simulink model "ExperimentalLab2Assignments"  (R2020b)
settings: Solver=VariableStepAuto  StartTime=0.0  StopTime=10.0  RelTol=1e-3
undefined symbols (not defined in the file): BEMF_Compensator, Beq_hat_final, C, denCd, DiscIntNeverNeededParam, friction_Compensator, Gamma0, gbox, H0, inertia_Compensator, J0, K, Kd, Ke, Ki, Kp, Kw, National_Instruments, Nu, numCd, Nx, PCIe, Phi0, rpm2rads, sens, stepAmplitude, tau_sf_hat_final, Tl, Ts
libraries: sldrtlib x15, simulink x1
settings Model: Creator=Musta  LastModifiedBy=Musta

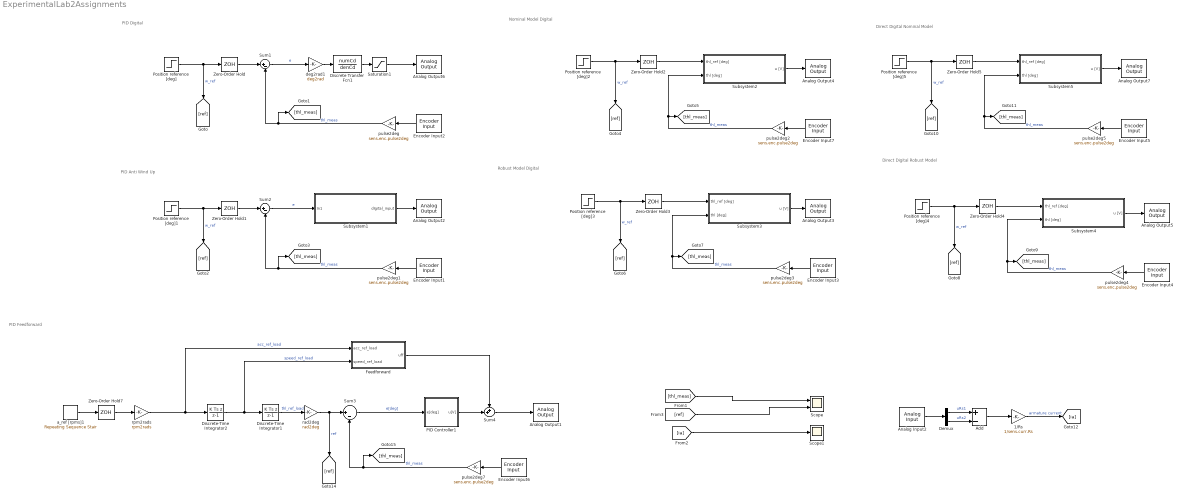
== system ExperimentalLab2Assignments ==
  note: PID Feedforward
  note: Direct Digital Nominal Model
  note: Direct Digital Robust Model
  note: Robust Model Digital
  note: Nominal Model Digital
  note: PID Anti Wind Up
  note: PID Digital
  1/Rs : Gain  Gain=1/sens.curr.Rs
  Add : Sum  Inputs=+-
  Analog Input2 : sldrtlib/Analog Input  SampleTime=0.001  MaxMissedTicks=10  ShowMissedTicks=off  YieldWhenWaiting=off  DrvName=National_Instruments/PCIe-6321  DrvAddress=4294967295  DrvOptions=[0 0 0 2 0 0 0]  Channels=[1,2]  RangeMode=1  VoltRange=1  DataType=1
      settings: AttributesFormatString=National Instruments\nPCIe-6321 [auto]
  Analog Output{1..7} (7 alike) : sldrtlib/Analog Output  SampleTime=0.001  MaxMissedTicks=10  ShowMissedTicks=off  YieldWhenWaiting=off  DrvName=National_Instruments/PCIe-6321  DrvAddress=4294967295  DrvOptions=[0 0 0 2 0 0 0]  Channels=1  RangeMode=1  VoltRange=1  InitialValue=0  FinalValue=0
      settings: AttributesFormatString=National Instruments\nPCIe-6321 [auto]
  Demux : Demux  Outputs=2
  Discrete Transfer Fcn1 : DiscreteTransferFcn  Numerator=numCd  Denominator=denCd  SampleTime=Ts
  Discrete-Time Integrator1 : DiscreteIntegrator  IntegratorMethod=Integration: Backward Euler  SampleTime=Ts  ICPrevOutput=DiscIntNeverNeededParam  ICPrevScaledInput=DiscIntNeverNeededParam
  Discrete-Time Integrator2 : DiscreteIntegrator  IntegratorMethod=Integration: Backward Euler  SampleTime=Ts  ICPrevOutput=DiscIntNeverNeededParam  ICPrevScaledInput=DiscIntNeverNeededParam
  Encoder Input{1..7} (7 alike) : sldrtlib/Encoder Input  SampleTime=0.001  MaxMissedTicks=10  ShowMissedTicks=off  YieldWhenWaiting=off  DrvName=National_Instruments/PCIe-6321  DrvAddress=4294967295  DrvOptions=[0 0 0 2 0 0 0]  Channels=1  QuadMode=3  IndexPulse=2  InputFilter=Inf  DataType=1
      settings: AttributesFormatString=National Instruments\nPCIe-6321 [auto]
  Feedforward : Subsystem
  PID Controller1 : Subsystem
  Position reference [deg]{,1..5} (6 alike) : Step  After=stepAmplitude  SampleTime=0
  Saturation1 : Saturate  UpperLimit=10  LowerLimit=-10
  Scope : Scope  NumInputPorts=2
  Scope1 : Scope
  Subsystem1 : Subsystem
  Subsystem2 : Subsystem
  Subsystem3 : Subsystem
  Subsystem4 : Subsystem
  Subsystem5 : Subsystem
  Sum1 : Sum  Inputs=|+-
  Sum2 : Sum  Inputs=|+-
  Sum3 : Sum  Inputs=|+-
  Sum4 : Sum  Inputs=++|
  Zero-Order Hold{,1..5,7} (7 alike) : ZeroOrderHold  SampleTime=Ts
  a_ref [rpms]1 : simulink/Sources/Repeating Sequence Stair  OutValues=[900 0 -900 -900 0 900].'  tsamp=0.5  OutMin=[]  OutMax=[]  OutDataTypeStr=double  OutputDataTypeScalingMode=double  OutDataType=fixdt(0,8)  ConRadixGroup=Best Precision: Vector-wise  OutScaling=2^-12
  deg2rad1 : Gain  Gain=deg2rad
  pulse2deg{,1..5,7} (7 alike) : Gain  Gain=sens.enc.pulse2deg
  rad2deg : Gain  Gain=rad2deg
  rpm2rads : Gain  Gain=rpm2rads
  wires:
  Zero-Order Hold/1 -> Sum1/1
  Saturation1/1 -> Analog Output6/1
  pulse2deg/1 -> [thl_meas], Sum1/2  "thl_meas"
  Position reference [deg]/1 -> Zero-Order Hold/1, [ref]  "w_ref"
  Encoder Input2/1 -> pulse2deg/1
  Sum1/1 -> deg2rad1/1  "e"
  Subsystem1/1(dIgital_input) -> Analog Output2/1
  Position reference [deg]1/1 -> Zero-Order Hold1/1, [ref]  "w_ref"
  Encoder Input1/1 -> pulse2deg1/1
  pulse2deg1/1 -> [thl_meas], Sum2/2  "thl_meas"
  Zero-Order Hold1/1 -> Sum2/1
  Sum2/1 -> Subsystem1/1(In1)  "e"
  Subsystem2/1(u [V]) -> Analog Output4/1
  Zero-Order Hold2/1 -> Subsystem2/1(thl_ref [deg])
  pulse2deg2/1 -> Subsystem2/2(thl [deg]), [thl_meas]  "thl_meas"
  Encoder Input7/1 -> pulse2deg2/1
  Position reference [deg]2/1 -> [ref], Zero-Order Hold2/1  "w_ref"
  Zero-Order Hold3/1 -> Subsystem3/1(thl_ref [deg])
  Position reference [deg]3/1 -> [ref], Zero-Order Hold3/1  "w_ref"
  Subsystem3/1(u [V]) -> Analog Output3/1
  Encoder Input3/1 -> pulse2deg3/1
  pulse2deg3/1 -> Subsystem3/2(thl [deg]), [thl_meas]  "thl_meas"
  Subsystem4/1(u [V]) -> Analog Output5/1
  Encoder Input4/1 -> pulse2deg4/1
  Position reference [deg]4/1 -> [ref], Zero-Order Hold4/1  "w_ref"
  pulse2deg4/1 -> Subsystem4/2(thl [deg]), [thl_meas]  "thl_meas"
  Zero-Order Hold4/1 -> Subsystem4/1(thl_ref [deg])
  Subsystem5/1(u [V]) -> Analog Output7/1
  Encoder Input5/1 -> pulse2deg5/1
  pulse2deg5/1 -> Subsystem5/2(thl [deg]), [thl_meas]  "thl_meas"
  Zero-Order Hold5/1 -> Subsystem5/1(thl_ref [deg])
  Position reference [deg]5/1 -> [ref], Zero-Order Hold5/1  "w_ref"
  Sum3/1 -> PID Controller1/1(e[deg])  "e[deg]"
  Discrete-Time Integrator2/1 -> Discrete-Time Integrator1/1, Feedforward/2(speed_ref_load)  "speed_ref_load"
  Zero-Order Hold7/1 -> rpm2rads/1
  Feedforward/1(uff) -> Sum4/1
  Discrete-Time Integrator1/1 -> rad2deg/1  "thl_ref_load"
  PID Controller1/1(u[V]) -> Sum4/2
  rad2deg/1 -> [ref], Sum3/1  "ref"
  rpm2rads/1 -> Discrete-Time Integrator2/1, Feedforward/1(acc_ref_load)  "acc_ref_load"
  a_ref [rpms]1/1 -> Zero-Order Hold7/1
  pulse2deg7/1 -> Sum3/2, [thl_meas]  "thl_meas"
  Encoder Input6/1 -> pulse2deg7/1
  Sum4/1 -> Analog Output1/1
  [thl_meas] -> Scope/1
  [ref] -> Scope/2
  [ia] -> Scope1/1
  Demux/2 -> Add/2  "uRs2"
  Analog Input2/1 -> Demux/1
  Add/1 -> 1/Rs/1
  Demux/1 -> Add/1  "uRs1"
  1/Rs/1 -> [ia]  "armature current"
  deg2rad1/1 -> Discrete Transfer Fcn1/1
  Discrete Transfer Fcn1/1 -> Saturation1/1

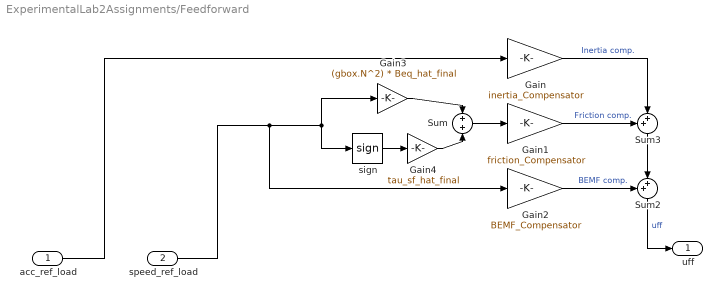
== system ExperimentalLab2Assignments/Feedforward ==
  acc_ref_load : Inport
  speed_ref_load : Inport  Port=2
  Gain : Gain  Gain=inertia_Compensator
  Gain1 : Gain  Gain=friction_Compensator
  Gain2 : Gain  Gain=BEMF_Compensator
  Gain3 : Gain  Gain=(gbox.N^2) * Beq_hat_final
  Gain4 : Gain  Gain=tau_sf_hat_final
  Sum : Sum  Inputs=+|+
  Sum2 : Sum  Inputs=++|
  Sum3 : Sum  Inputs=++|
  sign : Signum
  uff : Outport
  wires:
  sign/1 -> Gain4/1
  Sum/1 -> Gain1/1
  speed_ref_load/1 -> Gain2/1, sign/1, Gain3/1
  Sum3/1 -> Sum2/2
  Gain3/1 -> Sum/1
  Gain/1 -> Sum3/2  "Inertia comp."
  Gain1/1 -> Sum3/1  "Friction comp."
  Gain4/1 -> Sum/2
  Gain2/1 -> Sum2/1  "BEMF comp."
  acc_ref_load/1 -> Gain/1
  Sum2/1 -> uff/1  "uff"

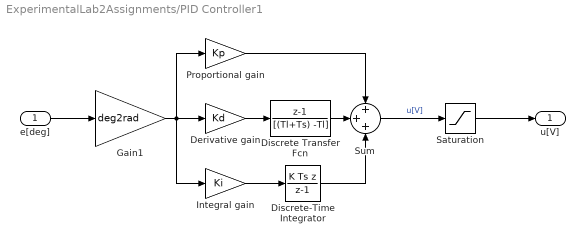
== system ExperimentalLab2Assignments/PID Controller1 ==
  e[deg] : Inport
  Derivative gain : Gain  Gain=Kd
  Discrete Transfer Fcn : DiscreteTransferFcn  Numerator=[1 -1]  Denominator=[(Tl+Ts) -Tl]  SampleTime=Ts
  Discrete-Time Integrator : DiscreteIntegrator  IntegratorMethod=Integration: Backward Euler  SampleTime=Ts  ICPrevOutput=DiscIntNeverNeededParam  ICPrevScaledInput=DiscIntNeverNeededParam
  Gain1 : Gain  Gain=deg2rad
  Integral gain : Gain  Gain=Ki
  Proportional gain : Gain  Gain=Kp
  Saturation : Saturate  UpperLimit=10  LowerLimit=-10
  Sum : Sum  Inputs=+++
  u[V] : Outport
  wires:
  e[deg]/1 -> Gain1/1
  Discrete Transfer Fcn/1 -> Sum/2
  Gain1/1 -> Proportional gain/1, Integral gain/1, Derivative gain/1
  Proportional gain/1 -> Sum/1
  Integral gain/1 -> Discrete-Time Integrator/1
  Discrete-Time Integrator/1 -> Sum/3
  Derivative gain/1 -> Discrete Transfer Fcn/1
  Sum/1 -> Saturation/1  "u[V]"
  Saturation/1 -> u[V]/1

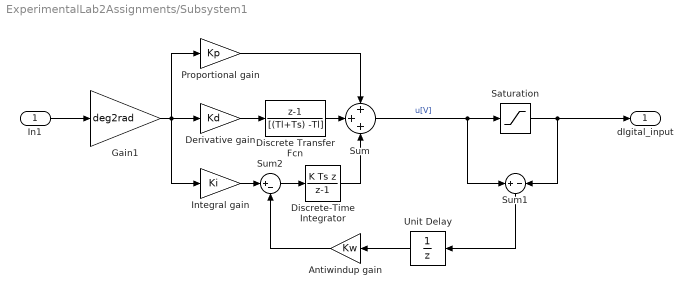
== system ExperimentalLab2Assignments/Subsystem1 ==
  In1 : Inport
  Antiwindup gain : Gain  Gain=Kw
  Derivative gain : Gain  Gain=Kd
  Discrete Transfer Fcn : DiscreteTransferFcn  Numerator=[1 -1]  Denominator=[(Tl+Ts) -Tl]  SampleTime=Ts
  Discrete-Time Integrator : DiscreteIntegrator  IntegratorMethod=Integration: Backward Euler  SampleTime=Ts  ICPrevOutput=DiscIntNeverNeededParam  ICPrevScaledInput=DiscIntNeverNeededParam
  Gain1 : Gain  Gain=deg2rad
  Integral gain : Gain  Gain=Ki
  Proportional gain : Gain  Gain=Kp
  Saturation : Saturate  UpperLimit=10  LowerLimit=-10
  Sum : Sum  Inputs=+++
  Sum1 : Sum  Inputs=+|-
  Sum2 : Sum  Inputs=|+-
  Unit Delay : UnitDelay  SampleTime=-1  HasFrameUpgradeWarning=on
  dIgital_input : Outport
  wires:
  Saturation/1 -> dIgital_input/1, Sum1/2
  Sum1/1 -> Unit Delay/1
  Unit Delay/1 -> Antiwindup gain/1
  Derivative gain/1 -> Discrete Transfer Fcn/1
  Gain1/1 -> Proportional gain/1, Integral gain/1, Derivative gain/1
  Discrete Transfer Fcn/1 -> Sum/2
  Discrete-Time Integrator/1 -> Sum/3
  In1/1 -> Gain1/1
  Integral gain/1 -> Sum2/1
  Sum/1 -> Sum1/1, Saturation/1  "u[V]"
  Proportional gain/1 -> Sum/1
  Antiwindup gain/1 -> Sum2/2
  Sum2/1 -> Discrete-Time Integrator/1

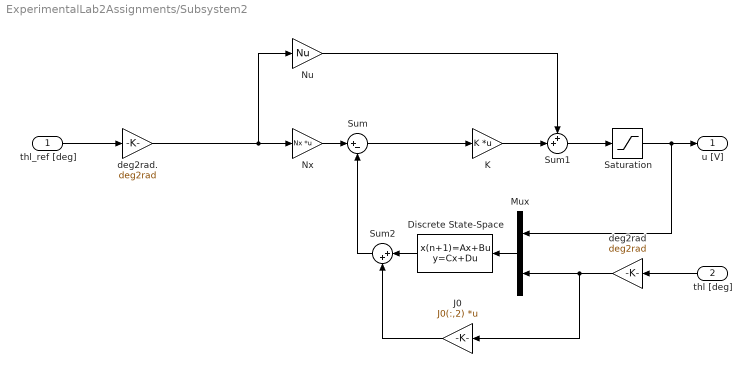
== system ExperimentalLab2Assignments/Subsystem2 ==
  thl_ref [deg] : Inport
  thl [deg] : Inport  Port=2
  Discrete State-Space : DiscreteStateSpace  A=Phi0  B=Gamma0  C=H0  D=zeros(size(H0,1),size(Gamma0,2))  SampleTime=Ts
  J0 : Gain  Gain=J0(:,2)  Multiplication=Matrix(K*u)
  K : Gain  Gain=K  Multiplication=Matrix(K*u)
  Mux : Mux  Inputs=2
  Nu : Gain  Gain=Nu
  Nx : Gain  Gain=Nx  Multiplication=Matrix(K*u)
  Saturation : Saturate  UpperLimit=10  LowerLimit=-10
  Sum : Sum  Inputs=|+-
  Sum1 : Sum  Inputs=++|
  Sum2 : Sum  Inputs=|++
  deg2rad : Gain  Gain=deg2rad
  deg2rad. : Gain  Gain=deg2rad
  u [V] : Outport
  wires:
  deg2rad/1 -> J0/1, Mux/2
  thl [deg]/1 -> deg2rad/1
  Saturation/1 -> Mux/1, u [V]/1
  thl_ref [deg]/1 -> deg2rad./1
  deg2rad./1 -> Nx/1, Nu/1
  Nx/1 -> Sum/1
  Mux/1 -> Discrete State-Space/1
  Sum/1 -> K/1
  K/1 -> Sum1/2
  Nu/1 -> Sum1/1
  Sum1/1 -> Saturation/1
  Discrete State-Space/1 -> Sum2/1
  J0/1 -> Sum2/2
  Sum2/1 -> Sum/2

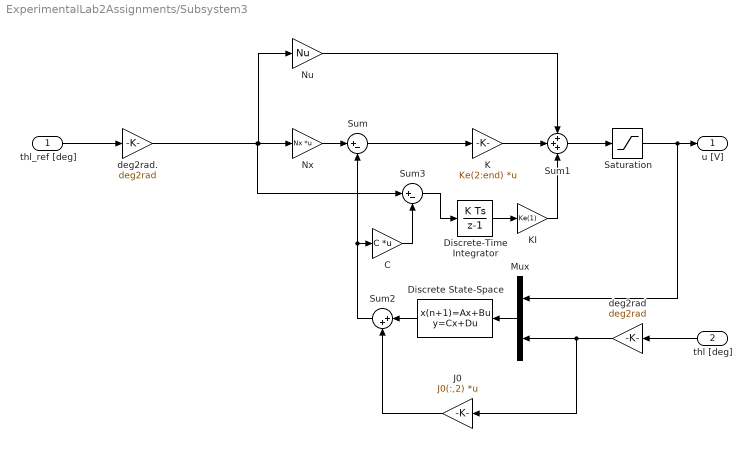
== system ExperimentalLab2Assignments/Subsystem3 ==
  thl_ref [deg] : Inport
  thl [deg] : Inport  Port=2
  C : Gain  Gain=C  Multiplication=Matrix(K*u)
  Discrete State-Space : DiscreteStateSpace  A=Phi0  B=Gamma0  C=H0  D=zeros(size(H0,1),size(Gamma0,2))  SampleTime=Ts
  Discrete-Time Integrator : DiscreteIntegrator  SampleTime=Ts  ICPrevOutput=DiscIntNeverNeededParam  ICPrevScaledInput=DiscIntNeverNeededParam
  J0 : Gain  Gain=J0(:,2)  Multiplication=Matrix(K*u)
  K : Gain  Gain=Ke(2:end)  Multiplication=Matrix(K*u)
  KI : Gain  Gain=Ke(1)
  Mux : Mux  Inputs=2
  Nu : Gain  Gain=Nu
  Nx : Gain  Gain=Nx  Multiplication=Matrix(K*u)
  Saturation : Saturate  UpperLimit=10  LowerLimit=-10
  Sum : Sum  Inputs=|+-
  Sum1 : Sum  Inputs=+++
  Sum2 : Sum  Inputs=|++
  Sum3 : Sum  Inputs=|+-
  deg2rad : Gain  Gain=deg2rad
  deg2rad. : Gain  Gain=deg2rad
  u [V] : Outport
  wires:
  deg2rad/1 -> J0/1, Mux/2
  thl [deg]/1 -> deg2rad/1
  Saturation/1 -> Mux/1, u [V]/1
  thl_ref [deg]/1 -> deg2rad./1
  Nx/1 -> Sum/1
  Mux/1 -> Discrete State-Space/1
  Sum/1 -> K/1
  K/1 -> Sum1/2
  Nu/1 -> Sum1/1
  Sum1/1 -> Saturation/1
  Discrete State-Space/1 -> Sum2/1
  J0/1 -> Sum2/2
  Sum2/1 -> Sum/2, C/1
  Discrete-Time Integrator/1 -> KI/1
  Sum3/1 -> Discrete-Time Integrator/1
  KI/1 -> Sum1/3
  deg2rad./1 -> Sum3/1, Nx/1, Nu/1
  C/1 -> Sum3/2

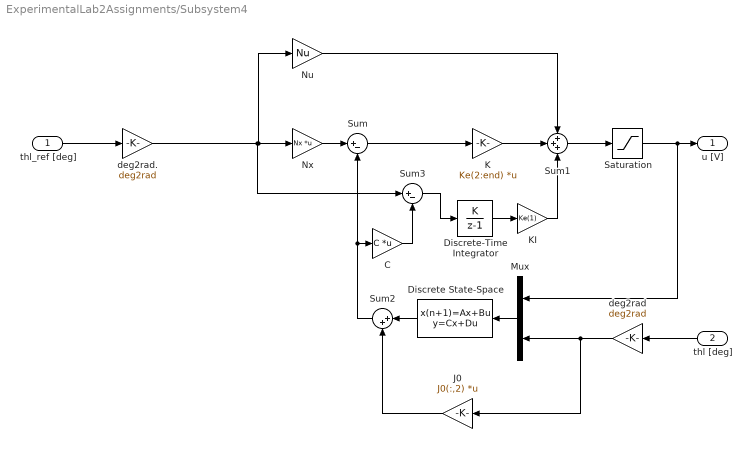
== system ExperimentalLab2Assignments/Subsystem4 ==
  thl_ref [deg] : Inport
  thl [deg] : Inport  Port=2
  C : Gain  Gain=C  Multiplication=Matrix(K*u)
  Discrete State-Space : DiscreteStateSpace  A=Phi0  B=Gamma0  C=H0  D=zeros(size(H0,1),size(Gamma0,2))  SampleTime=Ts
  Discrete-Time Integrator : DiscreteIntegrator  IntegratorMethod=Accumulation: Forward Euler  SampleTime=Ts  ICPrevOutput=DiscIntNeverNeededParam  ICPrevScaledInput=DiscIntNeverNeededParam
  J0 : Gain  Gain=J0(:,2)  Multiplication=Matrix(K*u)
  K : Gain  Gain=Ke(2:end)  Multiplication=Matrix(K*u)
  KI : Gain  Gain=Ke(1)
  Mux : Mux  Inputs=2
  Nu : Gain  Gain=Nu
  Nx : Gain  Gain=Nx  Multiplication=Matrix(K*u)
  Saturation : Saturate  UpperLimit=10  LowerLimit=-10
  Sum : Sum  Inputs=|+-
  Sum1 : Sum  Inputs=+++
  Sum2 : Sum  Inputs=|++
  Sum3 : Sum  Inputs=|+-
  deg2rad : Gain  Gain=deg2rad
  deg2rad. : Gain  Gain=deg2rad
  u [V] : Outport
  wires:
  deg2rad/1 -> J0/1, Mux/2
  thl [deg]/1 -> deg2rad/1
  Saturation/1 -> Mux/1, u [V]/1
  thl_ref [deg]/1 -> deg2rad./1
  Nx/1 -> Sum/1
  Mux/1 -> Discrete State-Space/1
  Sum/1 -> K/1
  K/1 -> Sum1/2
  Nu/1 -> Sum1/1
  Sum1/1 -> Saturation/1
  Discrete State-Space/1 -> Sum2/1
  J0/1 -> Sum2/2
  Sum2/1 -> Sum/2, C/1
  Discrete-Time Integrator/1 -> KI/1
  Sum3/1 -> Discrete-Time Integrator/1
  KI/1 -> Sum1/3
  deg2rad./1 -> Sum3/1, Nx/1, Nu/1
  C/1 -> Sum3/2

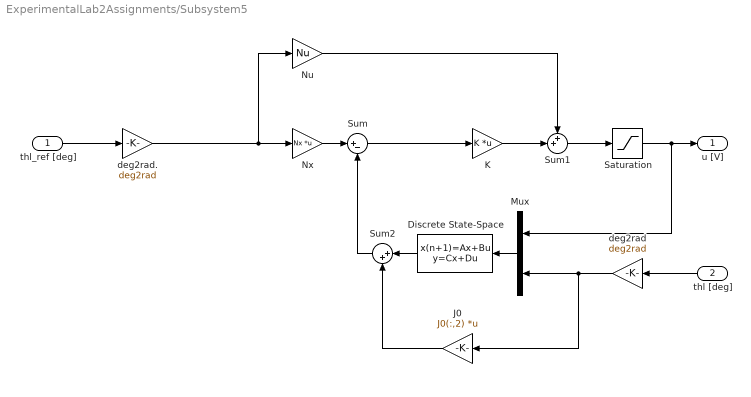
== system ExperimentalLab2Assignments/Subsystem5 ==
  thl_ref [deg] : Inport
  thl [deg] : Inport  Port=2
  Discrete State-Space : DiscreteStateSpace  A=Phi0  B=Gamma0  C=H0  D=zeros(size(H0,1),size(Gamma0,2))  SampleTime=Ts
  J0 : Gain  Gain=J0(:,2)  Multiplication=Matrix(K*u)
  K : Gain  Gain=K  Multiplication=Matrix(K*u)
  Mux : Mux  Inputs=2
  Nu : Gain  Gain=Nu
  Nx : Gain  Gain=Nx  Multiplication=Matrix(K*u)
  Saturation : Saturate  UpperLimit=10  LowerLimit=-10
  Sum : Sum  Inputs=|+-
  Sum1 : Sum  Inputs=++|
  Sum2 : Sum  Inputs=|++
  deg2rad : Gain  Gain=deg2rad
  deg2rad. : Gain  Gain=deg2rad
  u [V] : Outport
  wires:
  deg2rad/1 -> J0/1, Mux/2
  thl [deg]/1 -> deg2rad/1
  Saturation/1 -> Mux/1, u [V]/1
  thl_ref [deg]/1 -> deg2rad./1
  deg2rad./1 -> Nx/1, Nu/1
  Nx/1 -> Sum/1
  Mux/1 -> Discrete State-Space/1
  Sum/1 -> K/1
  K/1 -> Sum1/2
  Nu/1 -> Sum1/1
  Sum1/1 -> Saturation/1
  Discrete State-Space/1 -> Sum2/1
  J0/1 -> Sum2/2
  Sum2/1 -> Sum/2
